simulink model "ES008A_PwrSply"  (R2013b)
settings: Solver=FixedStepDiscrete  SolverMode=SingleTasking  StartTime=0.0  StopTime=1  FixedStep=0.002  RelTol=1e-3
values from neighbouring files (symbols this model uses):
  DiagcReg0Err = DataDict.NTC    [ES008A_PwrSply_DataDict.m]
  DiagcReg1Err = DataDict.NTC    [ES008A_PwrSply_DataDict.m]
  PWRSPLYDIAGREG0READVAL_CNT_U16 = DataDict.Constant    [ES008A_PwrSply_DataDict.m]
  PWRSPLYDIAGREG1READVAL_CNT_U16 = DataDict.Constant    [ES008A_PwrSply_DataDict.m]
  PwrSplyNtc0x07BFailStep = DataDict.Calibration    [ES008A_PwrSply_DataDict.m]
  PwrSplyNtc0x07BPassStep = DataDict.Calibration    [ES008A_PwrSply_DataDict.m]
  PwrSplyNtc0x07CFailStep = DataDict.Calibration    [ES008A_PwrSply_DataDict.m]
  PwrSplyNtc0x07CPassStep = DataDict.Calibration    [ES008A_PwrSply_DataDict.m]
  PwrSplyNtc0x07DFailStep = DataDict.Calibration    [ES008A_PwrSply_DataDict.m]
  PwrSplyNtc0x07DPassStep = DataDict.Calibration    [ES008A_PwrSply_DataDict.m]
  PWRSPLYOUTPENAWRVAL_CNT_U16 = DataDict.Constant    [ES008A_PwrSply_DataDict.m]
  PWRSPLYVRFYRESREG0READVAL_CNT_U16 = DataDict.Constant    [ES008A_PwrSply_DataDict.m]
  PWRSPLYVRFYRESREG1READVAL_CNT_U16 = DataDict.Constant    [ES008A_PwrSply_DataDict.m]
  SerlErr = DataDict.NTC    [ES008A_PwrSply_DataDict.m]
  SpiConf_SpiChannel_PwrSplyCh1 = DataDict.Constant    [ES008A_PwrSply_DataDict.m]
  SpiConf_SpiChannel_PwrSplyCh2 = DataDict.Constant    [ES008A_PwrSply_DataDict.m]
  SpiConf_SpiChannel_PwrSplyCh3 = DataDict.Constant    [ES008A_PwrSply_DataDict.m]
  SpiConf_SpiChannel_PwrSplyCh4 = DataDict.Constant    [ES008A_PwrSply_DataDict.m]
  SpiConf_SpiChannel_PwrSplyCh5 = DataDict.Constant    [ES008A_PwrSply_DataDict.m]
  SpiConf_SpiSequence_PwrSplySeq1 = DataDict.Constant    [ES008A_PwrSply_DataDict.m]
  SpiConf_SpiSequence_PwrSplySeq2 = DataDict.Constant    [ES008A_PwrSply_DataDict.m]
  SpiConf_SpiSequence_PwrSplySeq3 = DataDict.Constant    [ES008A_PwrSply_DataDict.m]
  SpiConf_SpiSequence_PwrSplySeq4 = DataDict.Constant    [ES008A_PwrSply_DataDict.m]
  SpiConf_SpiSequence_PwrSplySeq5 = DataDict.Constant    [ES008A_PwrSply_DataDict.m]
  StrtUpSelfTestReg0Err = DataDict.NTC    [ES008A_PwrSply_DataDict.m]
  StrtUpSelfTestReg1Err = DataDict.NTC    [ES008A_PwrSply_DataDict.m]
undefined symbols (not defined in the file or in its folder): sigbuilder_block, SysSt1
libraries: simulink x11
(part 4 of 4)

== stateflow chart ES008A_PwrSply/PwrSply/PwrSplyPer1/SysSt = Warm Init OR Enable/PwrSplyReadWrOrderFlg2 = 1 (Read Buffer)/Channel 4/No Startup Test Error 0/SetNtcSts/ISO Fault Debounce Design ==
  note: NTCSTS_PASSD           (0)
      | NTCSTS_FAILD             (1)
      | NTCSTS_PREPASSD   (2)
      | NTCSTS_PREFAILD     (3)
      |
      | SIGQLFR_NORES        (0)
      | SIGQLFR_PASSD         (1)
      | SIGQLFR_FAILD           (2)
  note: Pass Loop
  note: Fail Loop
  note: 
  (default) -> (junction 89)
  (junction 89) -> (junction 95) [order 1] : [NtcSts ==3]
  (junction 89) -> (junction 93) [order 2] : [NtcSts ==2]
  (junction 89) -> (junction 141) [order 3] : [NtcSts ==1]
      | { ErrAcc = 32767;
      | Qualifier =2;
      |  }
  (junction 89) -> (junction 141) [order 4] : [NtcSts ==0]
      | { ErrAcc = -32768;
      | Qualifier=1;
      | }
  (junction 95) -> (junction 103) [order 2]
  (junction 95) -> (junction 111) [order 1] : [ErrAcc <=0]
      | {ErrAcc = DebStep;}
  (junction 93) -> (junction 123) [order 2] : {
      | ErrAcc = ErrAcc - DebStep;
      | }
  (junction 93) -> (junction 123) [order 1] : [(ErrAcc - DebStep) <= -32768]
      | { ErrAcc = -32768;
      | Qualifier=1;
      | }
  (junction 103) -> (junction 111) [order 1] : [(ErrAcc + DebStep) <32767]
      | {ErrAcc = ErrAcc + DebStep;}
  (junction 103) -> (junction 111) [order 2] : {ErrAcc = 32767;
      | Qualifier =2;}
  (junction 123) -> (junction 141)
  (junction 111) -> (junction 141)
  (junction 141) -> (junction 159) [order 2] : {ErrAcc = 0;
      | Qualifier =0;
      | }
  (junction 141) -> (junction 159) [order 1] : [SvcClr ==0]
  data: NtcSts input uint8; Qualifier output uint8; DebStep input uint16; ErrAcc local int16; SvcClr input
